simulink model "three_phase_pwm_rectifier_ac_dc_model"  (R2019a)
settings: Solver=ode23t  StartTime=0.0  StopTime=10.0  MaxStep=1e-6  RelTol=1e-6
libraries: powerlib_meascontrol x1
settings Model: Creator=Görkem  LastModifiedBy=Görkem
settings DataIOCC: ReturnWorkspaceOutputs=off

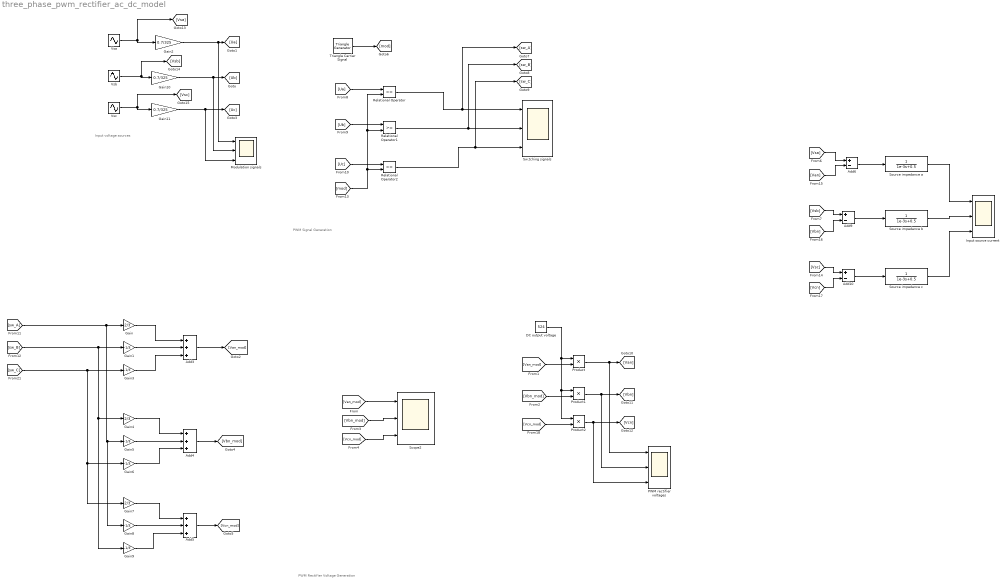
== system three_phase_pwm_rectifier_ac_dc_model ==
  note: PWM Rectifier Voltage Generation
  note: Input voltage sources
  note: PWM Signal Generation
  Add10 : Sum  Inputs=+-
  Add3 : Sum  Inputs=+++
  Add4 : Sum  Inputs=+++
  Add5 : Sum  Inputs=+++
  Add6 : Sum  Inputs=+-
  Add9 : Sum  Inputs=+-
  DC output voltage : Constant  Value=524
  Gain : Gain  Gain=2/3
  Gain{1,3,5..6,8..9} (6 alike) : Gain  Gain=-1/3
  Gain10 : Gain  Gain=0.7/325
  Gain11 : Gain  Gain=0.7/325
  Gain2 : Gain  Gain=0.7/325
  Gain4 : Gain  Gain=2/3
  Gain7 : Gain  Gain=2/3
  Input source current : Scope  NumInputPorts=3
  Modulation signals : Scope  NumInputPorts=3
  PWM rectifier voltages : Scope  NumInputPorts=3
  Product : Product
  Product1 : Product
  Product2 : Product
  Relational Operator : RelationalOperator  OutDataTypeStr=boolean  RndMeth=Simplest
  Relational Operator1 : RelationalOperator  OutDataTypeStr=boolean  RndMeth=Simplest
  Relational Operator2 : RelationalOperator  OutDataTypeStr=boolean  RndMeth=Simplest
  Scope2 : Scope  NumInputPorts=3
  Source impedance a : TransferFcn  Denominator=[1e-3 0.5]
  Source impedance b : TransferFcn  Denominator=[1e-3 0.5]
  Source impedance c : TransferFcn  Denominator=[1e-3 0.5]
  Sw,tching signals : Scope  NumInputPorts=3
  Triangle Carrier Signal : powerlib_meascontrol/Pulse & Signal Generators/Triangle Generator  Freq=10e3  Phase=-90  Ts=0
      settings: SourceProductName=Simscape Electrical
  Vsa : Sin  Amplitude=325  Frequency=2*pi*50  SampleTime=0
  Vsb : Sin  Amplitude=325  Frequency=2*pi*50  Phase=2*pi/3  SampleTime=0
  Vsc : Sin  Amplitude=325  Frequency=2*pi*50  Phase=4*pi/3  SampleTime=0
  wires:
  Gain/1 -> Add3/1
  Gain1/1 -> Add3/2
  Gain3/1 -> Add3/3
  Gain4/1 -> Add4/1
  Gain5/1 -> Add4/2
  Gain6/1 -> Add4/3
  Gain7/1 -> Add5/1
  Gain8/1 -> Add5/2
  Gain9/1 -> Add5/3
  Add4/1 -> [Vbn_mod]
  [Van_mod] -> Product/2
  DC output voltage/1 -> Product2/1, Product1/1, Product/1
  [Vbn_mod] -> Product1/2
  [Vcn_mod] -> Product2/2
  [sw_A] -> Gain8/1, Gain5/1, Gain/1
  [sw_B] -> Gain9/1, Gain4/1, Gain1/1
  [sw_C] -> Gain7/1, Gain6/1, Gain3/1
  Add3/1 -> [Van_mod]
  Add5/1 -> [Vcn_mod]
  Gain11/1 -> Modulation signals/3, [Uc]
  Gain2/1 -> Modulation signals/1, [Ua]
  Gain10/1 -> Modulation signals/2, [Ub]
  Relational Operator2/1 -> [sw_C], Sw,tching signals/3
  Relational Operator1/1 -> [sw_B], Sw,tching signals/2
  Relational Operator/1 -> [sw_A], Sw,tching signals/1
  Triangle Carrier Signal/1 -> [mod]
  Vsc/1 -> Gain11/1, [Vsc]
  Vsb/1 -> Gain10/1, [Vsb]
  Vsa/1 -> Gain2/1, [Vsa]
  Product/1 -> PWM rectifier voltages/1, [Van]
  Product1/1 -> PWM rectifier voltages/2, [Vbn]
  Product2/1 -> PWM rectifier voltages/3, [Vcn]
  [Van_mod] -> Scope2/1
  [Vbn_mod] -> Scope2/2
  [Vcn_mod] -> Scope2/3
  [Vsa] -> Add6/1
  [Van] -> Add6/2
  [Vsb] -> Add9/1
  [Vbn] -> Add9/2
  [Vsc] -> Add10/1
  [Vcn] -> Add10/2
  Source impedance b/1 -> Input source current/2
  Source impedance c/1 -> Input source current/3
  Source impedance a/1 -> Input source current/1
  Add6/1 -> Source impedance a/1
  Add9/1 -> Source impedance b/1
  Add10/1 -> Source impedance c/1
  [Ua] -> Relational Operator/1
  [Ub] -> Relational Operator1/1
  [Uc] -> Relational Operator2/1
  [mod] -> Relational Operator2/2, Relational Operator1/2, Relational Operator/2
